simulink model "full_correlator"  (R2022a)
settings: Solver=VariableStepDiscrete  StartTime=0.0  StopTime=4000  RelTol=1e-3
libraries: hdlBasic x2638, hdlSSR x215, hdlDSPIP x4, xbsIndex_r4 x1, xps_library x1
(part 3 of 43)

== system full_correlator/Subsystem ==
  din : Inport
  vin : Inport  Port=2
  Concat : hdlBasic/Concat  num_inputs=8  XmcBlockStatus=1  maskContainerNames=group1  block_type=concat  block_config=sysgen:Concat_config
  Reinterpret : hdlBasic/Reinterpret  force_arith_type=on  arith_type=Unsigned  force_bin_pt=on  bin_pt=0  XmcBlockStatus=1  maskContainerNames=group1  block_type=reinterpret  block_config=sysgen:Reinterpret_config
  Scalar to Vector2 : hdlSSR/Scalar2Vector  Width=18  sg_ssr=8  block_type=scalar2vector_ssr  XmcBlockStatus=1  sg_ssr_prev=8  maskContainerNames=group1
  Time Division Demultiplexer2 : hdlBasic/Time Division Demultiplexer  frame_pattern=[1 1 1 1 1 1 1 1]  impl_style=Multiple Channel  vin=on  explicit_period=off  period=1  XmcBlockStatus=1  maskContainerNames=group2  block_type=tdd  block_config=sysgen:TDD_config
  Vector Reinterpret2 : hdlSSR/Vector Reinterpret  force_arith_type=on  arith_type="Signed  (2's comp)"  force_bin_pt=on  bin_pt=17  sg_ssr=8  block_type=reinterpret_ssr  XmcBlockStatus=1  sg_ssr_prev=8  maskContainerNames=group1
  dout : Outport
  vout : Outport  Port=2
  wires:
  Time Division Demultiplexer2/8 -> Concat/1
  Time Division Demultiplexer2/5 -> Concat/4
  Time Division Demultiplexer2/9 -> vout/1
  din/1 -> Reinterpret/1
  Time Division Demultiplexer2/3 -> Concat/6
  Reinterpret/1 -> Time Division Demultiplexer2/1
  Scalar to Vector2/1 -> Vector Reinterpret2/1
  Time Division Demultiplexer2/6 -> Concat/3
  Concat/1 -> Scalar to Vector2/1
  Time Division Demultiplexer2/7 -> Concat/2
  Time Division Demultiplexer2/4 -> Concat/5
  Time Division Demultiplexer2/2 -> Concat/7
  Vector Reinterpret2/1 -> dout/1
  vin/1 -> Time Division Demultiplexer2/2
  Time Division Demultiplexer2/1 -> Concat/8

== system full_correlator/Subsystem1 ==
  addr : Inport
  we : Inport  Port=2
  din : Inport  Port=3
  Concat{,1..3} (4 alike) : hdlBasic/Concat  num_inputs=2  XmcBlockStatus=1  maskContainerNames=group1  block_type=concat  block_config=sysgen:Concat_config
  Constant{2..5} (4 alike) : hdlBasic/Constant  const=0  gui_display_data_type=Fixed-point  arith_type=Unsigned  n_bits=56  bin_pt=0  preci_type=Single  exp_width=8  frac_width=24  explicit_period=off  period=1  XmcBlockStatus=1  maskContainerNames=tabcontainer1  block_type=constant  block_config=sysgen:Constant_config
  Terminator{7..10} (4 alike) : Terminator
  Vector Reinterpret : hdlSSR/Vector Reinterpret  force_arith_type=on  arith_type=Unsigned  force_bin_pt=on  bin_pt=0  sg_ssr=16  block_type=reinterpret_ssr  XmcBlockStatus=1  sg_ssr_prev=16  maskContainerNames=group1
  Vector to Scalar : hdlSSR/Vector2Scalar  sg_ssr=16  block_type=vector2scalar_ssr  XmcBlockStatus=1  sg_ssr_prev=16  maskContainerNames=group1
  bus_expand : Subsystem  AncestorBlock=casper_library_flow_control/bus_expand  mask(bus_expand){mode=divisions of equal size, outputNum=4, outputWidth=72, outputBinaryPt=0, outputArithmeticType=0, show_format=off, outputToWorkspace=off, variablePrefix=out, outputToModelAsWell=on}
      mask prompts: outputNum "Number of outputs:"; outputWidth "Output width:"; outputBinaryPt "Output binary point position:"; outputArithmeticType "Output arithmetic type (ufix=0, fix=1, bool=2):"; show_format "Print format string?"; outputToWorkspace "Output to workspace?"; variablePrefix "Variable name prefix:"; outputToModelAsWell "Output to model as well?"
      mask help:
      | Expands a 'bus' made using a bus_create or Xilinx
      | concat block.
      | The input will be divided into the specified number
      | of outputs with the specified arithmetic types.
      | Divisions are made from most significant bit.
      mask init: same as full_correlator/bus_expand
      settings: AttributesFormatString=4 outputs
      mask TypeOptions mode: divisions of equal size | divisions of arbitrary size
      mask Callback mode: %bus_expand_callback();
      mask Callback outputWidth: %bus_expand_callback();
      mask Callback outputToWorkspace: %bus_expand_callback();
  shared_bram : Subsystem  Tag=xps:bram  AncestorBlock=xps_library/Memory/shared_bram  mask{arith_type=Unsigned, addr_width=6, data_width=128, reg_prim_output=off, reg_core_output=off, optimization=Minimum_Area, data_bin_pt=0, init_vals=[0:2^10-1], sample_rate=1}
      mask prompts: arith_type "Output Data Type"; addr_width "Address width"; data_width "Data Width"; reg_prim_output "Register Primitive Output"; reg_core_output "Register Core Output"; data_bin_pt "Data Binary Point"; init_vals "Initial values (simulation only)"; sample_rate "Sample rate"
      mask init:
      | shared_bram_mask;
      mask TypeOptions arith_type: Unsigned | Signed  (2's comp)
      mask TypeOptions data_width: 8 | 16 | 32 | 64 | 128
      mask TypeOptions optimization: Minimum_Area | Low_Power
  shared_bram1 : Subsystem  Tag=xps:bram  AncestorBlock=xps_library/Memory/shared_bram  mask{arith_type=Unsigned, addr_width=6, data_width=128, reg_prim_output=off, reg_core_output=off, optimization=Minimum_Area, data_bin_pt=0, init_vals=[0:2^10-1], sample_rate=1}
      mask prompts: arith_type "Output Data Type"; addr_width "Address width"; data_width "Data Width"; reg_prim_output "Register Primitive Output"; reg_core_output "Register Core Output"; data_bin_pt "Data Binary Point"; init_vals "Initial values (simulation only)"; sample_rate "Sample rate"
      mask init:
      | shared_bram_mask;
      mask TypeOptions arith_type: Unsigned | Signed  (2's comp)
      mask TypeOptions data_width: 8 | 16 | 32 | 64 | 128
      mask TypeOptions optimization: Minimum_Area | Low_Power
  shared_bram2 : Subsystem  Tag=xps:bram  AncestorBlock=xps_library/Memory/shared_bram  mask{arith_type=Unsigned, addr_width=6, data_width=128, reg_prim_output=off, reg_core_output=off, optimization=Minimum_Area, data_bin_pt=0, init_vals=[0:2^10-1], sample_rate=1}
      mask prompts: arith_type "Output Data Type"; addr_width "Address width"; data_width "Data Width"; reg_prim_output "Register Primitive Output"; reg_core_output "Register Core Output"; data_bin_pt "Data Binary Point"; init_vals "Initial values (simulation only)"; sample_rate "Sample rate"
      mask init:
      | shared_bram_mask;
      mask TypeOptions arith_type: Unsigned | Signed  (2's comp)
      mask TypeOptions data_width: 8 | 16 | 32 | 64 | 128
      mask TypeOptions optimization: Minimum_Area | Low_Power
  shared_bram3 : Subsystem  Tag=xps:bram  AncestorBlock=xps_library/Memory/shared_bram  mask{arith_type=Unsigned, addr_width=6, data_width=128, reg_prim_output=off, reg_core_output=off, optimization=Minimum_Area, data_bin_pt=0, init_vals=[0:2^10-1], sample_rate=1}
      mask prompts: arith_type "Output Data Type"; addr_width "Address width"; data_width "Data Width"; reg_prim_output "Register Primitive Output"; reg_core_output "Register Core Output"; data_bin_pt "Data Binary Point"; init_vals "Initial values (simulation only)"; sample_rate "Sample rate"
      mask init:
      | shared_bram_mask;
      mask TypeOptions arith_type: Unsigned | Signed  (2's comp)
      mask TypeOptions data_width: 8 | 16 | 32 | 64 | 128
      mask TypeOptions optimization: Minimum_Area | Low_Power
  wires:
  Constant3/1 -> Concat1/2
  shared_bram1/1(data_out) -> Terminator8/1
  Constant5/1 -> Concat3/2
  addr/1 -> shared_bram/1(addr), shared_bram1/1(addr), shared_bram2/1(addr), shared_bram3/1(addr)
  shared_bram/1(data_out) -> Terminator7/1
  Constant2/1 -> Concat/2
  shared_bram3/1(data_out) -> Terminator10/1
  Concat1/1 -> shared_bram1/2(data_in)
  Constant4/1 -> Concat2/2
  din/1 -> Vector Reinterpret/1
  shared_bram2/1(data_out) -> Terminator9/1
  we/1 -> shared_bram/3(we), shared_bram1/3(we), shared_bram2/3(we), shared_bram3/3(we)
  Concat3/1 -> shared_bram3/2(data_in)
  Concat/1 -> shared_bram/2(data_in)
  Concat2/1 -> shared_bram2/2(data_in)
  Vector Reinterpret/1 -> Vector to Scalar/1
  Vector to Scalar/1 -> bus_expand/1(bus_in)
  bus_expand/1(msb_out4) -> Concat/1
  bus_expand/2(out3) -> Concat1/1
  bus_expand/3(out2) -> Concat2/1
  bus_expand/4(lsb_out1) -> Concat3/1

== system full_correlator/Subsystem2 ==
  addr : Inport
  we : Inport  Port=2
  din : Inport  Port=3
  Concat{,1..3} (4 alike) : hdlBasic/Concat  num_inputs=2  XmcBlockStatus=1  maskContainerNames=group1  block_type=concat  block_config=sysgen:Concat_config
  Constant{2..5} (4 alike) : hdlBasic/Constant  const=0  gui_display_data_type=Fixed-point  arith_type=Unsigned  n_bits=56  bin_pt=0  preci_type=Single  exp_width=8  frac_width=24  explicit_period=off  period=1  XmcBlockStatus=1  maskContainerNames=tabcontainer1  block_type=constant  block_config=sysgen:Constant_config
  Terminator{7..10} (4 alike) : Terminator
  Vector Reinterpret : hdlSSR/Vector Reinterpret  force_arith_type=on  arith_type=Unsigned  force_bin_pt=on  bin_pt=0  sg_ssr=16  block_type=reinterpret_ssr  XmcBlockStatus=1  sg_ssr_prev=16  maskContainerNames=group1
  Vector to Scalar : hdlSSR/Vector2Scalar  sg_ssr=16  block_type=vector2scalar_ssr  XmcBlockStatus=1  sg_ssr_prev=16  maskContainerNames=group1
  bus_expand : Subsystem  AncestorBlock=casper_library_flow_control/bus_expand  mask(bus_expand){mode=divisions of equal size, outputNum=4, outputWidth=72, outputBinaryPt=0, outputArithmeticType=0, show_format=off, outputToWorkspace=off, variablePrefix=out, outputToModelAsWell=on}
      mask prompts: outputNum "Number of outputs:"; outputWidth "Output width:"; outputBinaryPt "Output binary point position:"; outputArithmeticType "Output arithmetic type (ufix=0, fix=1, bool=2):"; show_format "Print format string?"; outputToWorkspace "Output to workspace?"; variablePrefix "Variable name prefix:"; outputToModelAsWell "Output to model as well?"
      mask help:
      | Expands a 'bus' made using a bus_create or Xilinx
      | concat block.
      | The input will be divided into the specified number
      | of outputs with the specified arithmetic types.
      | Divisions are made from most significant bit.
      mask init: same as full_correlator/bus_expand
      settings: AttributesFormatString=4 outputs
      mask TypeOptions mode: divisions of equal size | divisions of arbitrary size
      mask Callback mode: %bus_expand_callback();
      mask Callback outputWidth: %bus_expand_callback();
      mask Callback outputToWorkspace: %bus_expand_callback();
  shared_bram : Subsystem  Tag=xps:bram  AncestorBlock=xps_library/Memory/shared_bram  mask{arith_type=Unsigned, addr_width=6, data_width=128, reg_prim_output=off, reg_core_output=off, optimization=Minimum_Area, data_bin_pt=0, init_vals=[0:2^10-1], sample_rate=1}
      mask prompts: arith_type "Output Data Type"; addr_width "Address width"; data_width "Data Width"; reg_prim_output "Register Primitive Output"; reg_core_output "Register Core Output"; data_bin_pt "Data Binary Point"; init_vals "Initial values (simulation only)"; sample_rate "Sample rate"
      mask init:
      | shared_bram_mask;
      mask TypeOptions arith_type: Unsigned | Signed  (2's comp)
      mask TypeOptions data_width: 8 | 16 | 32 | 64 | 128
      mask TypeOptions optimization: Minimum_Area | Low_Power
  shared_bram1 : Subsystem  Tag=xps:bram  AncestorBlock=xps_library/Memory/shared_bram  mask{arith_type=Unsigned, addr_width=6, data_width=128, reg_prim_output=off, reg_core_output=off, optimization=Minimum_Area, data_bin_pt=0, init_vals=[0:2^10-1], sample_rate=1}
      mask prompts: arith_type "Output Data Type"; addr_width "Address width"; data_width "Data Width"; reg_prim_output "Register Primitive Output"; reg_core_output "Register Core Output"; data_bin_pt "Data Binary Point"; init_vals "Initial values (simulation only)"; sample_rate "Sample rate"
      mask init:
      | shared_bram_mask;
      mask TypeOptions arith_type: Unsigned | Signed  (2's comp)
      mask TypeOptions data_width: 8 | 16 | 32 | 64 | 128
      mask TypeOptions optimization: Minimum_Area | Low_Power
  shared_bram2 : Subsystem  Tag=xps:bram  AncestorBlock=xps_library/Memory/shared_bram  mask{arith_type=Unsigned, addr_width=6, data_width=128, reg_prim_output=off, reg_core_output=off, optimization=Minimum_Area, data_bin_pt=0, init_vals=[0:2^10-1], sample_rate=1}
      mask prompts: arith_type "Output Data Type"; addr_width "Address width"; data_width "Data Width"; reg_prim_output "Register Primitive Output"; reg_core_output "Register Core Output"; data_bin_pt "Data Binary Point"; init_vals "Initial values (simulation only)"; sample_rate "Sample rate"
      mask init:
      | shared_bram_mask;
      mask TypeOptions arith_type: Unsigned | Signed  (2's comp)
      mask TypeOptions data_width: 8 | 16 | 32 | 64 | 128
      mask TypeOptions optimization: Minimum_Area | Low_Power
  shared_bram3 : Subsystem  Tag=xps:bram  AncestorBlock=xps_library/Memory/shared_bram  mask{arith_type=Unsigned, addr_width=6, data_width=128, reg_prim_output=off, reg_core_output=off, optimization=Minimum_Area, data_bin_pt=0, init_vals=[0:2^10-1], sample_rate=1}
      mask prompts: arith_type "Output Data Type"; addr_width "Address width"; data_width "Data Width"; reg_prim_output "Register Primitive Output"; reg_core_output "Register Core Output"; data_bin_pt "Data Binary Point"; init_vals "Initial values (simulation only)"; sample_rate "Sample rate"
      mask init:
      | shared_bram_mask;
      mask TypeOptions arith_type: Unsigned | Signed  (2's comp)
      mask TypeOptions data_width: 8 | 16 | 32 | 64 | 128
      mask TypeOptions optimization: Minimum_Area | Low_Power
  wires:
  Constant3/1 -> Concat1/2
  shared_bram1/1(data_out) -> Terminator8/1
  Constant5/1 -> Concat3/2
  addr/1 -> shared_bram/1(addr), shared_bram1/1(addr), shared_bram2/1(addr), shared_bram3/1(addr)
  shared_bram/1(data_out) -> Terminator7/1
  Constant2/1 -> Concat/2
  shared_bram3/1(data_out) -> Terminator10/1
  Concat1/1 -> shared_bram1/2(data_in)
  Constant4/1 -> Concat2/2
  din/1 -> Vector Reinterpret/1
  shared_bram2/1(data_out) -> Terminator9/1
  we/1 -> shared_bram/3(we), shared_bram1/3(we), shared_bram2/3(we), shared_bram3/3(we)
  Concat3/1 -> shared_bram3/2(data_in)
  Concat/1 -> shared_bram/2(data_in)
  Concat2/1 -> shared_bram2/2(data_in)
  Vector Reinterpret/1 -> Vector to Scalar/1
  Vector to Scalar/1 -> bus_expand/1(bus_in)
  bus_expand/1(msb_out4) -> Concat/1
  bus_expand/2(out3) -> Concat1/1
  bus_expand/3(out2) -> Concat2/1
  bus_expand/4(lsb_out1) -> Concat3/1

== system full_correlator/Subsystem3 ==
  din : Inport
  vin : Inport  Port=2
  Concat : hdlBasic/Concat  num_inputs=8  XmcBlockStatus=1  maskContainerNames=group1  block_type=concat  block_config=sysgen:Concat_config
  Reinterpret : hdlBasic/Reinterpret  force_arith_type=on  arith_type=Unsigned  force_bin_pt=on  bin_pt=0  XmcBlockStatus=1  maskContainerNames=group1  block_type=reinterpret  block_config=sysgen:Reinterpret_config
  Scalar to Vector2 : hdlSSR/Scalar2Vector  Width=18  sg_ssr=8  block_type=scalar2vector_ssr  XmcBlockStatus=1  sg_ssr_prev=8  maskContainerNames=group1
  Time Division Demultiplexer2 : hdlBasic/Time Division Demultiplexer  frame_pattern=[1 1 1 1 1 1 1 1]  impl_style=Multiple Channel  vin=on  explicit_period=off  period=1  XmcBlockStatus=1  maskContainerNames=group2  block_type=tdd  block_config=sysgen:TDD_config
  Vector Reinterpret2 : hdlSSR/Vector Reinterpret  force_arith_type=on  arith_type="Signed  (2's comp)"  force_bin_pt=on  bin_pt=17  sg_ssr=8  block_type=reinterpret_ssr  XmcBlockStatus=1  sg_ssr_prev=8  maskContainerNames=group1
  dout : Outport
  vout : Outport  Port=2
  wires:
  Time Division Demultiplexer2/8 -> Concat/1
  Time Division Demultiplexer2/5 -> Concat/4
  Time Division Demultiplexer2/9 -> vout/1
  din/1 -> Reinterpret/1
  Time Division Demultiplexer2/3 -> Concat/6
  Reinterpret/1 -> Time Division Demultiplexer2/1
  Scalar to Vector2/1 -> Vector Reinterpret2/1
  Time Division Demultiplexer2/6 -> Concat/3
  Concat/1 -> Scalar to Vector2/1
  Time Division Demultiplexer2/7 -> Concat/2
  Time Division Demultiplexer2/4 -> Concat/5
  Time Division Demultiplexer2/2 -> Concat/7
  Vector Reinterpret2/1 -> dout/1
  vin/1 -> Time Division Demultiplexer2/2
  Time Division Demultiplexer2/1 -> Concat/8

== system full_correlator/Subsystem4 ==
  IN : Inport
  Scalar to Vector2 : hdlSSR/Scalar2Vector  Width=18  sg_ssr=8  block_type=scalar2vector_ssr  XmcBlockStatus=1  sg_ssr_prev=8  maskContainerNames=group1
  Up Sample2 : hdlBasic/Up Sample  sample_ratio=8  copy_samples=on  en=off  latency=1  XmcBlockStatus=1  maskContainerNames=group1  block_type=usamp  block_config=sysgen:Upsample_config
  Vector Reinterpret2 : hdlSSR/Vector Reinterpret  force_arith_type=on  arith_type=Unsigned  force_bin_pt=on  bin_pt=0  sg_ssr=8  block_type=reinterpret_ssr  XmcBlockStatus=1  sg_ssr_prev=8  maskContainerNames=group1
  Vector Reinterpret3 : hdlSSR/Vector Reinterpret  force_arith_type=on  arith_type="Signed  (2's comp)"  force_bin_pt=on  bin_pt=17  sg_ssr=8  block_type=reinterpret_ssr  XmcBlockStatus=1  sg_ssr_prev=8  maskContainerNames=group1
  Vector to Scalar1 : hdlSSR/Vector2Scalar  sg_ssr=8  block_type=vector2scalar_ssr  XmcBlockStatus=1  sg_ssr_prev=8  maskContainerNames=group1
  OUT : Outport
  wires:
  Scalar to Vector2/1 -> Vector Reinterpret3/1
  Vector Reinterpret3/1 -> OUT/1
  Vector Reinterpret2/1 -> Vector to Scalar1/1
  Vector to Scalar1/1 -> Up Sample2/1
  Up Sample2/1 -> Scalar to Vector2/1
  IN/1 -> Vector Reinterpret2/1

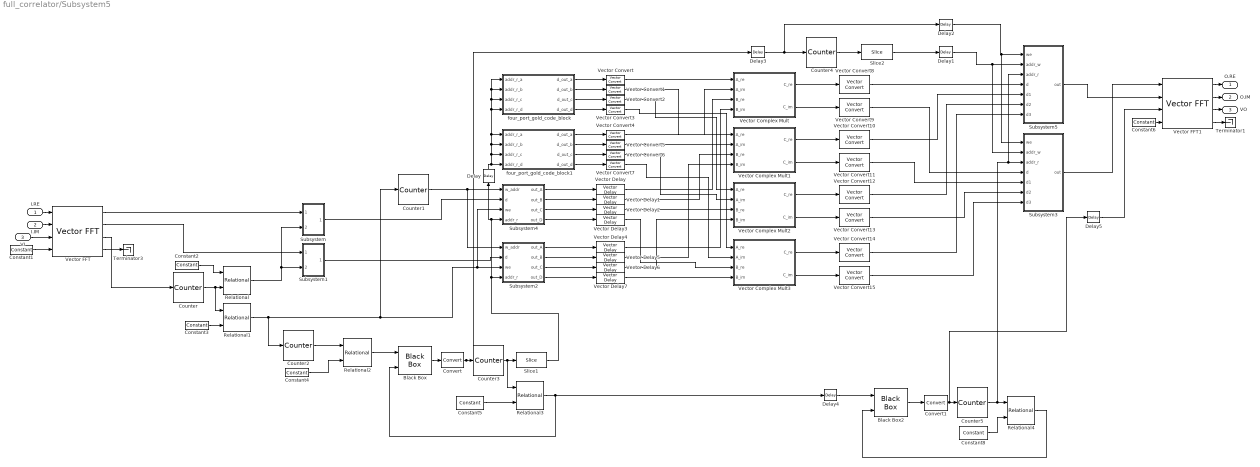
== system full_correlator/Subsystem5 ==
  I.RE : Inport
  I.IM : Inport  Port=2
  VI : Inport  Port=3
  Black Box : hdlBasic/Black Box  init_code=sr_flip_flop_config  sim_method=Vivado Simulator  verbose=off  XmcBlockStatus=1  maskContainerNames=group1  block_type=blackbox2  block_config=sysgen:black_box_config
  Black Box2 : hdlBasic/Black Box  init_code=sr_flip_flop_config  sim_method=Vivado Simulator  verbose=off  XmcBlockStatus=1  maskContainerNames=group1  block_type=blackbox2  block_config=sysgen:black_box_config
  Constant1 : hdlBasic/Constant  const=1023  gui_display_data_type=Fixed-point  arith_type=Unsigned  n_bits=10  bin_pt=0  preci_type=Single  exp_width=8  frac_width=24  explicit_period=on  period=1  XmcBlockStatus=1  maskContainerNames=tabcontainer1  block_type=constant  block_config=sysgen:Constant_config
  Constant2 : hdlBasic/Constant  const=0  gui_display_data_type=Fixed-point  arith_type=Unsigned  n_bits=1  bin_pt=0  preci_type=Single  exp_width=8  frac_width=24  explicit_period=on  period=1  XmcBlockStatus=1  maskContainerNames=tabcontainer1  block_type=constant  block_config=sysgen:Constant_config
  Constant3 : hdlBasic/Constant  const=1  gui_display_data_type=Fixed-point  arith_type=Unsigned  n_bits=1  bin_pt=0  preci_type=Single  exp_width=8  frac_width=24  explicit_period=on  period=1  XmcBlockStatus=1  maskContainerNames=tabcontainer1  block_type=constant  block_config=sysgen:Constant_config
  Constant4 : hdlBasic/Constant  const=63  gui_display_data_type=Fixed-point  arith_type=Unsigned  n_bits=6  bin_pt=0  preci_type=Single  exp_width=8  frac_width=24  explicit_period=on  period=1  XmcBlockStatus=1  maskContainerNames=tabcontainer1  block_type=constant  block_config=sysgen:Constant_config
  Constant5 : hdlBasic/Constant  const=126  gui_display_data_type=Fixed-point  arith_type=Unsigned  n_bits=7  bin_pt=0  preci_type=Single  exp_width=8  frac_width=24  explicit_period=on  period=1  XmcBlockStatus=1  maskContainerNames=tabcontainer1  block_type=constant  block_config=sysgen:Constant_config
  Constant6 : hdlBasic/Constant  const=1023  gui_display_data_type=Fixed-point  arith_type=Unsigned  n_bits=10  bin_pt=0  preci_type=Single  exp_width=8  frac_width=24  explicit_period=on  period=1  XmcBlockStatus=1  maskContainerNames=tabcontainer1  block_type=constant  block_config=sysgen:Constant_config
  Constant8 : hdlBasic/Constant  const=62  gui_display_data_type=Fixed-point  arith_type=Unsigned  n_bits=6  bin_pt=0  preci_type=Single  exp_width=8  frac_width=24  explicit_period=on  period=1  XmcBlockStatus=1  maskContainerNames=tabcontainer1  block_type=constant  block_config=sysgen:Constant_config
  Convert : hdlBasic/Convert  gui_display_data_type=Boolean  arith_type=Boolean  n_bits=16  bin_pt=14  float_type=Single  exp_bits=8  fraction_bits=24  quantization=Truncate  overflow=Wrap  en=off  latency=0  pipeline=off  XmcBlockStatus=1  maskContainerNames=group2  block_type=convert  block_config=sysgen:Convert_config  block_width=595  block_height=885
  Convert1 : hdlBasic/Convert  gui_display_data_type=Boolean  arith_type=Boolean  n_bits=16  bin_pt=14  float_type=Single  exp_bits=8  fraction_bits=24  quantization=Truncate  overflow=Wrap  en=off  latency=0  pipeline=off  XmcBlockStatus=1  maskContainerNames=group2  block_type=convert  block_config=sysgen:Convert_config  block_width=595  block_height=885
  Counter : hdlBasic/Counter  cnt_type=Free running  cnt_to=Inf  operation=Up  start_count=0  cnt_by_val=1  arith_type=Unsigned  n_bits=1  bin_pt=0  load_pin=off  rst=off  en=on  explicit_period=Explicit  period=1  use_behavioral_HDL=off  implementation=Fabric  XmcBlockStatus=1  maskContainerNames=group1  block_type=counter  block_config=sysgen:Counter_config  block_width=531  block_height=1023
  Counter1 : hdlBasic/Counter  cnt_type=Free running  cnt_to=Inf  operation=Up  start_count=0  cnt_by_val=1  arith_type=Unsigned  n_bits=6  bin_pt=0  load_pin=off  rst=off  en=on  explicit_period=Explicit  period=1  use_behavioral_HDL=off  implementation=Fabric  XmcBlockStatus=1  maskContainerNames=group1  block_type=counter  block_config=sysgen:Counter_config  block_width=531  block_height=1023
  Counter2 : hdlBasic/Counter  cnt_type=Free running  cnt_to=Inf  operation=Up  start_count=0  cnt_by_val=1  arith_type=Unsigned  n_bits=6  bin_pt=0  load_pin=off  rst=off  en=on  explicit_period=Explicit  period=1  use_behavioral_HDL=off  implementation=Fabric  XmcBlockStatus=1  maskContainerNames=group1  block_type=counter  block_config=sysgen:Counter_config  block_width=531  block_height=1023
  Counter3 : hdlBasic/Counter  cnt_type=Free running  cnt_to=Inf  operation=Up  start_count=0  cnt_by_val=1  arith_type=Unsigned  n_bits=7  bin_pt=0  load_pin=off  rst=off  en=on  explicit_period=Explicit  period=1  use_behavioral_HDL=off  implementation=Fabric  XmcBlockStatus=1  maskContainerNames=group1  block_type=counter  block_config=sysgen:Counter_config  block_width=531  block_height=1023
  Counter4 : hdlBasic/Counter  cnt_type=Free running  cnt_to=Inf  operation=Up  start_count=0  cnt_by_val=1  arith_type=Unsigned  n_bits=7  bin_pt=0  load_pin=off  rst=off  en=on  explicit_period=Explicit  period=1  use_behavioral_HDL=off  implementation=Fabric  XmcBlockStatus=1  maskContainerNames=group1  block_type=counter  block_config=sysgen:Counter_config  block_width=531  block_height=1023
  Counter5 : hdlBasic/Counter  cnt_type=Free running  cnt_to=Inf  operation=Up  start_count=0  cnt_by_val=1  arith_type=Unsigned  n_bits=6  bin_pt=0  load_pin=off  rst=off  en=on  explicit_period=Explicit  period=1  use_behavioral_HDL=off  implementation=Fabric  XmcBlockStatus=1  maskContainerNames=group1  block_type=counter  block_config=sysgen:Counter_config  block_width=531  block_height=1023
  Delay : hdlBasic/Delay  rst=off  en=off  latency=2  reg_retiming=off  XmcBlockStatus=1  maskContainerNames=group1  block_type=delay  block_config=sysgen:Delay_config
  Delay1 : hdlBasic/Delay  rst=off  en=off  latency=1  reg_retiming=off  XmcBlockStatus=1  maskContainerNames=group1  block_type=delay  block_config=sysgen:Delay_config
  Delay2 : hdlBasic/Delay  rst=off  en=off  latency=1  reg_retiming=off  XmcBlockStatus=1  maskContainerNames=group1  block_type=delay  block_config=sysgen:Delay_config
  Delay3 : hdlBasic/Delay  rst=off  en=off  latency=10  reg_retiming=off  XmcBlockStatus=1  maskContainerNames=group1  block_type=delay  block_config=sysgen:Delay_config
  Delay4 : hdlBasic/Delay  rst=off  en=off  latency=11  reg_retiming=off  XmcBlockStatus=1  maskContainerNames=group1  block_type=delay  block_config=sysgen:Delay_config
  Delay5 : hdlBasic/Delay  rst=off  en=off  latency=6  reg_retiming=off  XmcBlockStatus=1  maskContainerNames=group1  block_type=delay  block_config=sysgen:Delay_config
  Relational : hdlBasic/Relational  mode=a=b  op_type=Bool  en=off  latency=0  XmcBlockStatus=1  maskContainerNames=tabcontainer1  block_type=relational  block_config=sysgen:Relational_config
  Relational1 : hdlBasic/Relational  mode=a=b  op_type=Bool  en=off  latency=0  XmcBlockStatus=1  maskContainerNames=tabcontainer1  block_type=relational  block_config=sysgen:Relational_config
  Relational2 : hdlBasic/Relational  mode=a=b  op_type=Bool  en=off  latency=1  XmcBlockStatus=1  maskContainerNames=tabcontainer1  block_type=relational  block_config=sysgen:Relational_config
  Relational3 : hdlBasic/Relational  mode=a=b  op_type=Bool  en=off  latency=1  XmcBlockStatus=1  maskContainerNames=tabcontainer1  block_type=relational  block_config=sysgen:Relational_config
  Relational4 : hdlBasic/Relational  mode=a=b  op_type=Bool  en=off  latency=1  XmcBlockStatus=1  maskContainerNames=tabcontainer1  block_type=relational  block_config=sysgen:Relational_config
  Slice1 : hdlBasic/Slice  nbits=4  boolean_output=off  mode=Upper Bit Location + Width  bit1=0  base1=MSB of Input  bit0=0  base0=LSB of Input  XmcBlockStatus=1  maskContainerNames=group1  block_type=slice  block_config=sysgen:Slice_config
  Slice2 : hdlBasic/Slice  nbits=4  boolean_output=off  mode=Upper Bit Location + Width  bit1=0  base1=MSB of Input  bit0=0  base0=LSB of Input  XmcBlockStatus=1  maskContainerNames=group1  block_type=slice  block_config=sysgen:Slice_config
  Subsystem : Subsystem
  Subsystem1 : Subsystem
  Subsystem2 : Subsystem
  Subsystem3 : Subsystem
  Subsystem4 : Subsystem
  Subsystem5 : Subsystem
  Terminator1 : Terminator
  Terminator3 : Terminator
  Vector Complex Mult : Subsystem  LoadFcn=obj = XmcLoadGUI(gcbh); obj.loadGUI();  mask(Xilinx Vector Complex Multiplier Block){sg_ssr=16, use_synth_mdl=off, sg_icon_stat=, sg_mask_display=|, block_version=, block_type=cmplxmult_ssr, XmcBlockStatus=1, sg_ssr_prev=16, SD={'sg_ssr'=>'Int','use_synth_mdl'=>'Int','xinports'=>'DoubleVector','xoutports'=>'DoubleVector','block_type'=>'String'}, maskContainerNames=group1}
      mask sg_mask_display=|
      | xmcDrawHDLBlockIcon();
      | fprintf('','COMMENT: begin icon text');
      |
      | color('black');port_label('input',1,' A_re');
      | color('black');port_label('input',2,' A_im');
      | color('black');port_label('input',3,' B_re');
      | color('black');port_label('input',4,' B_im');
      |
      | color('black');disp('25x18 signed \newline Latency = 6','texmode','on');
      |
      | color('black');port_label('output',1,'C_re');
      | color('black');port_label('output',2,'C_im');
      mask prompts: sg_ssr "SSR"; use_synth_mdl "Use Synthesizable model"
      mask help: Vector Complex Multiplier block supports complext multiplication for input of vector types.
      mask init:
      | this = gcb;
      | xlSSRParamEvaluation;
      | isElabReq = xlSSRIsElabReq(this,sg_ssr);
      | if (sg_ssr ~= sg_ssr_prev || isElabReq)
      |     try
      |         xlSSRCmplxMult;
      |         set_param(this,'sg_ssr_prev',num2str(sg_ssr));
      |     catch ME
      |         disp(['Error while updating -> ' this])
      |         disp(ME.message)
      |     end
      | else
      |    xlSSRCmplxMultInitGUI;
      | end
      mask Help: helpview(vmcHelp)
      mask Callback sg_ssr: obj = XmcUpdateGUI(gcbh, @xlmagicenablement, -1); obj.updateGUI()
      mask Callback use_synth_mdl: obj = XmcUpdateGUI(gcbh, @xlmagicenablement, -1); obj.updateGUI()
      mask TypeOptions maskContainerNames: group1 | infoedit | tabcontainer1 | basictab | Impltab
      mask DialogControl DescGroupVar Prompt: Vector Complex Mult
      mask DialogControl infoedit Prompt: The Vector Complex Multiplier block supports multiplication of two complex input vectors.
      mask DialogControl basictab Prompt: Basic
      mask DialogControl Impltab Prompt: Implementation
      mask Display:
      | xmcDrawHDLBlockIcon();
      | fprintf('','COMMENT: begin icon text');
      | 
      | color('black');port_label('input',1,' A_re');
      | color('black');port_label('input',2,' A_im');
      | color('black');port_label('input',3,' B_re');
      | color('black');port_label('input',4,' B_im');
      | 
      | color('black');disp('25x18 signed \newline Latency = 6','texmode','on');
      | 
      | color('black');port_label('output',1,'C_re');
      | color('black');port_label('output',2,'C_im');
  Vector Complex Mult1 : Subsystem  LoadFcn=obj = XmcLoadGUI(gcbh); obj.loadGUI();  mask(Xilinx Vector Complex Multiplier Block){sg_ssr=16, use_synth_mdl=off, sg_icon_stat=, sg_mask_display=|, block_version=, block_type=cmplxmult_ssr, XmcBlockStatus=1, sg_ssr_prev=16, SD={'sg_ssr'=>'Int','use_synth_mdl'=>'Int','xinports'=>'DoubleVector','xoutports'=>'DoubleVector','block_type'=>'String'}, maskContainerNames=group1}
      mask sg_mask_display=|
      | xmcDrawHDLBlockIcon();
      | fprintf('','COMMENT: begin icon text');
      |
      | color('black');port_label('input',1,' A_re');
      | color('black');port_label('input',2,' A_im');
      | color('black');port_label('input',3,' B_re');
      | color('black');port_label('input',4,' B_im');
      |
      | color('black');disp('25x18 signed \newline Latency = 6','texmode','on');
      |
      | color('black');port_label('output',1,'C_re');
      | color('black');port_label('output',2,'C_im');
      mask prompts: sg_ssr "SSR"; use_synth_mdl "Use Synthesizable model"
      mask help: Vector Complex Multiplier block supports complext multiplication for input of vector types.
      mask init: same as full_correlator/Subsystem5/Vector Complex Mult
      mask Help: helpview(vmcHelp)
      mask Callback sg_ssr: obj = XmcUpdateGUI(gcbh, @xlmagicenablement, -1); obj.updateGUI()
      mask Callback use_synth_mdl: obj = XmcUpdateGUI(gcbh, @xlmagicenablement, -1); obj.updateGUI()
      mask TypeOptions maskContainerNames: group1 | infoedit | tabcontainer1 | basictab | Impltab
      mask DialogControl DescGroupVar Prompt: Vector Complex Mult
      mask DialogControl infoedit Prompt: The Vector Complex Multiplier block supports multiplication of two complex input vectors.
      mask DialogControl basictab Prompt: Basic
      mask DialogControl Impltab Prompt: Implementation
      mask Display:
      | xmcDrawHDLBlockIcon();
      | fprintf('','COMMENT: begin icon text');
      | 
      | color('black');port_label('input',1,' A_re');
      | color('black');port_label('input',2,' A_im');
      | color('black');port_label('input',3,' B_re');
      | color('black');port_label('input',4,' B_im');
      | 
      | color('black');disp('25x18 signed \newline Latency = 6','texmode','on');
      | 
      | color('black');port_label('output',1,'C_re');
      | color('black');port_label('output',2,'C_im');
  Vector Complex Mult2 : Subsystem  LoadFcn=obj = XmcLoadGUI(gcbh); obj.loadGUI();  mask(Xilinx Vector Complex Multiplier Block){sg_ssr=16, use_synth_mdl=off, sg_icon_stat=, sg_mask_display=|, block_version=, block_type=cmplxmult_ssr, XmcBlockStatus=1, sg_ssr_prev=16, SD={'sg_ssr'=>'Int','use_synth_mdl'=>'Int','xinports'=>'DoubleVector','xoutports'=>'DoubleVector','block_type'=>'String'}, maskContainerNames=group1}
      mask sg_mask_display=|
      | xmcDrawHDLBlockIcon();
      | fprintf('','COMMENT: begin icon text');
      |
      | color('black');port_label('input',1,' A_re');
      | color('black');port_label('input',2,' A_im');
      | color('black');port_label('input',3,' B_re');
      | color('black');port_label('input',4,' B_im');
      |
      | color('black');disp('25x18 signed \newline Latency = 6','texmode','on');
      |
      | color('black');port_label('output',1,'C_re');
      | color('black');port_label('output',2,'C_im');
      mask prompts: sg_ssr "SSR"; use_synth_mdl "Use Synthesizable model"
      mask help: Vector Complex Multiplier block supports complext multiplication for input of vector types.
      mask init: same as full_correlator/Subsystem5/Vector Complex Mult
      mask Help: helpview(vmcHelp)
      mask Callback sg_ssr: obj = XmcUpdateGUI(gcbh, @xlmagicenablement, -1); obj.updateGUI()
      mask Callback use_synth_mdl: obj = XmcUpdateGUI(gcbh, @xlmagicenablement, -1); obj.updateGUI()
      mask TypeOptions maskContainerNames: group1 | infoedit | tabcontainer1 | basictab | Impltab
      mask DialogControl DescGroupVar Prompt: Vector Complex Mult
      mask DialogControl infoedit Prompt: The Vector Complex Multiplier block supports multiplication of two complex input vectors.
      mask DialogControl basictab Prompt: Basic
      mask DialogControl Impltab Prompt: Implementation
      mask Display:
      | xmcDrawHDLBlockIcon();
      | fprintf('','COMMENT: begin icon text');
      | 
      | color('black');port_label('input',1,' A_re');
      | color('black');port_label('input',2,' A_im');
      | color('black');port_label('input',3,' B_re');
      | color('black');port_label('input',4,' B_im');
      | 
      | color('black');disp('25x18 signed \newline Latency = 6','texmode','on');
      | 
      | color('black');port_label('output',1,'C_re');
      | color('black');port_label('output',2,'C_im');
  Vector Complex Mult3 : Subsystem  LoadFcn=obj = XmcLoadGUI(gcbh); obj.loadGUI();  mask(Xilinx Vector Complex Multiplier Block){sg_ssr=16, use_synth_mdl=off, sg_icon_stat=, sg_mask_display=|, block_version=, block_type=cmplxmult_ssr, XmcBlockStatus=1, sg_ssr_prev=16, SD={'sg_ssr'=>'Int','use_synth_mdl'=>'Int','xinports'=>'DoubleVector','xoutports'=>'DoubleVector','block_type'=>'String'}, maskContainerNames=group1}
      mask sg_mask_display=|
      | xmcDrawHDLBlockIcon();
      | fprintf('','COMMENT: begin icon text');
      |
      | color('black');port_label('input',1,' A_re');
      | color('black');port_label('input',2,' A_im');
      | color('black');port_label('input',3,' B_re');
      | color('black');port_label('input',4,' B_im');
      |
      | color('black');disp('25x18 signed \newline Latency = 6','texmode','on');
      |
      | color('black');port_label('output',1,'C_re');
      | color('black');port_label('output',2,'C_im');
      mask prompts: sg_ssr "SSR"; use_synth_mdl "Use Synthesizable model"
      mask help: Vector Complex Multiplier block supports complext multiplication for input of vector types.
      mask init: same as full_correlator/Subsystem5/Vector Complex Mult
      mask Help: helpview(vmcHelp)
      mask Callback sg_ssr: obj = XmcUpdateGUI(gcbh, @xlmagicenablement, -1); obj.updateGUI()
      mask Callback use_synth_mdl: obj = XmcUpdateGUI(gcbh, @xlmagicenablement, -1); obj.updateGUI()
      mask TypeOptions maskContainerNames: group1 | infoedit | tabcontainer1 | basictab | Impltab
      mask DialogControl DescGroupVar Prompt: Vector Complex Mult
      mask DialogControl infoedit Prompt: The Vector Complex Multiplier block supports multiplication of two complex input vectors.
      mask DialogControl basictab Prompt: Basic
      mask DialogControl Impltab Prompt: Implementation
      mask Display:
      | xmcDrawHDLBlockIcon();
      | fprintf('','COMMENT: begin icon text');
      | 
      | color('black');port_label('input',1,' A_re');
      | color('black');port_label('input',2,' A_im');
      | color('black');port_label('input',3,' B_re');
      | color('black');port_label('input',4,' B_im');
      | 
      | color('black');disp('25x18 signed \newline Latency = 6','texmode','on');
      | 
      | color('black');port_label('output',1,'C_re');
      | color('black');port_label('output',2,'C_im');
  Vector Convert{,1..7} (8 alike) : hdlSSR/Vector Convert  gui_display_data_type=Fixed-point  arith_type=Signed (2's comp)  n_bits=26  bin_pt=17  float_type=Single  exp_bits=8  fraction_bits=24  quantization=Truncate  overflow=Wrap  en=off  sg_latency=1  sg_ssr=16  pipeline=off  block_type=convert_ssr  XmcBlockStatus=1  sg_ssr_prev=16  maskContainerNames=group2
  Vector Convert{8..15} (8 alike) : hdlSSR/Vector Convert  gui_display_data_type=Fixed-point  arith_type=Signed (2's comp)  n_bits=18  bin_pt=17  float_type=Single  exp_bits=8  fraction_bits=24  quantization=Truncate  overflow=Wrap  en=off  sg_latency=1  sg_ssr=16  pipeline=off  block_type=convert_ssr  XmcBlockStatus=1  sg_ssr_prev=16  maskContainerNames=group2
  Vector Delay{,1..7} (8 alike) : hdlSSR/Vector Delay  rst=off  en=off  vectorize_en=off  sg_latency=1  sg_ssr=16  reg_retiming=off  block_type=delay_ssr  XmcBlockStatus=1  sg_ssr_prev=16  maskContainerNames=group1
  Vector FFT : hdlSSR/Vector FFT  N=1024  n_bits=18  bin_pt=17  bram_threshold=258  sg_ssr=8  block_type=fft_ssr  W_high=1  W_low=-17  XmcBlockStatus=1  sg_ssr_prev=8  maskContainerNames=group3
  Vector FFT1 : hdlSSR/Vector FFT  N=1024  n_bits=18  bin_pt=17  bram_threshold=258  sg_ssr=16  block_type=fft_ssr  W_high=1  W_low=-17  XmcBlockStatus=1  sg_ssr_prev=16  maskContainerNames=group3
  four_port_gold_code_block : Subsystem
  four_port_gold_code_block1 : Subsystem
  O.RE : Outport
  O.IM : Outport  Port=2
  VO : Outport  Port=3
  wires:
  Subsystem5/1(out) -> Vector FFT1/2
  Subsystem2/3(out_C) -> Vector Delay6/1
  Vector Complex Mult1/1(C_re) -> Vector Convert10/1
  Black Box2/1 -> Convert1/1
  Vector Delay5/1 -> Vector Complex Mult1/4(B_im)
  Vector Complex Mult2/1(C_re) -> Vector Convert12/1
  Vector Convert9/1 -> Subsystem3/4(d)
  Vector Convert/1 -> Vector Complex Mult/1(A_re)
  Vector Convert15/1 -> Subsystem3/7(d3)
  Vector Convert14/1 -> Subsystem5/7(d3)
  Subsystem2/2(out_B) -> Vector Delay5/1
  Vector Convert13/1 -> Subsystem3/6(d2)
  Vector FFT1/4 -> Terminator1/1
  Subsystem4/2(out_B) -> Vector Delay1/1
  Delay2/1 -> Subsystem5/1(we), Subsystem3/1(we)
  Vector Convert8/1 -> Subsystem5/4(d)
  Vector Complex Mult/1(C_re) -> Vector Convert8/1
  Vector Complex Mult/2(C_im) -> Vector Convert9/1
  Delay4/1 -> Black Box2/1
  Vector Delay1/1 -> Vector Complex Mult1/3(B_re)
  Vector FFT/1 -> Subsystem/1(din)
  four_port_gold_code_block/3(d_out_c) -> Vector Convert2/1
  four_port_gold_code_block1/1(d_out_a) -> Vector Convert4/1
  VI/1 -> Vector FFT/3
  Vector Complex Mult2/2(C_im) -> Vector Convert13/1
  Vector Complex Mult3/2(C_im) -> Vector Convert15/1
  Vector Convert11/1 -> Subsystem3/5(d1)
  Vector Delay2/1 -> Vector Complex Mult2/3(B_re)
  Subsystem/1(out) -> Subsystem4/2(d)
  Vector Complex Mult3/1(C_re) -> Vector Convert14/1
  Subsystem4/3(out_C) -> Vector Delay2/1
  Relational3/1 -> Black Box/2, Delay4/1
  Delay5/1 -> Vector FFT1/3
  Constant8/1 -> Relational4/2
  Relational2/1 -> Black Box/1
  Vector Convert1/1 -> Vector Complex Mult1/1(A_re)
  Vector Delay6/1 -> Vector Complex Mult2/4(B_im)
  Counter3/1 -> Slice1/1, Relational3/1
  Subsystem2/1(out_A) -> Vector Delay4/1
  Delay3/1 -> Delay2/1, Counter4/1
  Vector Complex Mult1/2(C_im) -> Vector Convert11/1
  Vector Delay4/1 -> Vector Complex Mult/4(B_im)
  Delay/1 -> four_port_gold_code_block1/4(addr_r_d), four_port_gold_code_block1/3(addr_r_c), four_port_gold_code_block1/2(addr_r_b), four_port_gold_code_block1/1(addr_r_a), four_port_gold_code_block/4(addr_r_d), four_port_gold_code_block/3(addr_r_c), four_port_gold_code_block/2(addr_r_b), four_port_gold_code_block/1(addr_r_a)
  Vector FFT1/2 -> O.IM/1
  Convert/1 -> Delay3/1, Counter3/1
  I.IM/1 -> Vector FFT/2
  Vector Delay/1 -> Vector Complex Mult/3(B_re)
  four_port_gold_code_block/1(d_out_a) -> Vector Convert/1
  Subsystem2/4(out_D) -> Vector Delay7/1
  Vector FFT1/3 -> VO/1
  Vector Convert5/1 -> Vector Complex Mult1/2(A_im)
  Constant3/1 -> Relational1/2
  Vector FFT/2 -> Subsystem1/1(din)
  Vector FFT1/1 -> O.RE/1
  Counter5/1 -> Subsystem5/3(addr_r), Subsystem3/3(addr_r), Relational4/1
  Vector Delay3/1 -> Vector Complex Mult3/3(B_re)
  four_port_gold_code_block1/4(d_out_d) -> Vector Convert7/1
  Counter1/1 -> Subsystem2/1(w_addr), Subsystem4/1(w_addr)
  Vector Delay7/1 -> Vector Complex Mult3/4(B_im)
  Subsystem4/4(out_D) -> Vector Delay3/1
  Black Box/1 -> Convert/1
  Delay1/1 -> Subsystem5/2(addr_w), Subsystem3/2(addr_w)
  Vector FFT/4 -> Terminator3/1
  Vector Convert12/1 -> Subsystem5/6(d2)
  Vector FFT/3 -> Counter/1
  Relational1/1 -> Subsystem2/3(we), Subsystem4/3(we), Counter1/1, Counter2/1
  Constant6/1 -> Vector FFT1/4
  four_port_gold_code_block1/2(d_out_b) -> Vector Convert5/1
  Constant2/1 -> Relational/1
  Vector Convert2/1 -> Vector Complex Mult2/1(A_re)
  Constant4/1 -> Relational2/2
  Convert1/1 -> Delay5/1, Counter5/1
  Counter4/1 -> Slice2/1
  Vector Convert7/1 -> Vector Complex Mult3/2(A_im)
  Relational4/1 -> Black Box2/2
  Relational/1 -> Subsystem1/2(hold), Subsystem/2(hold)
  Vector Convert6/1 -> Vector Complex Mult2/2(A_im)
  Slice2/1 -> Delay1/1
  four_port_gold_code_block/2(d_out_b) -> Vector Convert1/1
  Vector Convert10/1 -> Subsystem5/5(d1)
  Constant5/1 -> Relational3/2
  Vector Convert3/1 -> Vector Complex Mult3/1(A_re)
  four_port_gold_code_block1/3(d_out_c) -> Vector Convert6/1
  Slice1/1 -> Subsystem2/4(addr_r), Delay/1, Subsystem4/4(addr_r)
  Counter/1 -> Relational1/1, Relational/2
  Subsystem3/1(out) -> Vector FFT1/1
  I.RE/1 -> Vector FFT/1
  Constant1/1 -> Vector FFT/4
  Subsystem1/1(out) -> Subsystem2/2(d)
  four_port_gold_code_block/4(d_out_d) -> Vector Convert3/1
  Vector Convert4/1 -> Vector Complex Mult/2(A_im)
  Counter2/1 -> Relational2/1
  Subsystem4/1(out_A) -> Vector Delay/1

== system full_correlator/Subsystem6 ==
  IN : Inport
  Scalar to Vector2 : hdlSSR/Scalar2Vector  Width=18  sg_ssr=8  block_type=scalar2vector_ssr  XmcBlockStatus=1  sg_ssr_prev=8  maskContainerNames=group1
  Up Sample2 : hdlBasic/Up Sample  sample_ratio=8  copy_samples=on  en=off  latency=1  XmcBlockStatus=1  maskContainerNames=group1  block_type=usamp  block_config=sysgen:Upsample_config
  Vector Reinterpret2 : hdlSSR/Vector Reinterpret  force_arith_type=on  arith_type=Unsigned  force_bin_pt=on  bin_pt=0  sg_ssr=8  block_type=reinterpret_ssr  XmcBlockStatus=1  sg_ssr_prev=8  maskContainerNames=group1
  Vector Reinterpret3 : hdlSSR/Vector Reinterpret  force_arith_type=on  arith_type="Signed  (2's comp)"  force_bin_pt=on  bin_pt=17  sg_ssr=8  block_type=reinterpret_ssr  XmcBlockStatus=1  sg_ssr_prev=8  maskContainerNames=group1
  Vector to Scalar1 : hdlSSR/Vector2Scalar  sg_ssr=8  block_type=vector2scalar_ssr  XmcBlockStatus=1  sg_ssr_prev=8  maskContainerNames=group1
  OUT : Outport
  wires:
  Scalar to Vector2/1 -> Vector Reinterpret3/1
  Vector Reinterpret3/1 -> OUT/1
  Vector Reinterpret2/1 -> Vector to Scalar1/1
  Vector to Scalar1/1 -> Up Sample2/1
  Up Sample2/1 -> Scalar to Vector2/1
  IN/1 -> Vector Reinterpret2/1

== system full_correlator/adc_real_stream ==
  out_reg : Inport
  assert_reg : hdlBasic/Assert  assert_type=on  type_source=Explicitly  gui_display_data_type=Fixed-point  arith_type=Unsigned  n_bits=16  bin_pt=0  preci_type=Single  exp_width=8  frac_width=24  assert_rate=off  rate_source=Explicitly  period=1  output_port=on  XmcBlockStatus=0  maskContainerNames=group1  block_type=assert  block_config=sysgen:assert_config  block_width=609  block_height=900
  cast_gw : hdlBasic/Convert  gui_display_data_type=Fixed-point  arith_type=Unsigned  n_bits=32  bin_pt=0  float_type=Single  exp_bits=8  fraction_bits=24  quantization=Truncate  overflow=Wrap  en=off  latency=1  pipeline=off  XmcBlockStatus=0  maskContainerNames=group2  block_type=convert  block_config=sysgen:Convert_config  block_width=595  block_height=885
  full_correlator_adc_real_stream_user_data_in : hdlBasic/Gateway Out  inherit_from_input=off  hdl_port=on  rows=1  columns=1  UseAsDAC=off  DACChannel='1'  interface=None  automatic_assignment=on  address_offset=hex2dec('00')  intf_name=''  intf_description=''  timing_constraint=None  locs_specified=off  LOCs={}  io_standard={}  XmcBlockStatus=0  maskContainerNames=group4  block_type=gatewayout  block_config=sysgen:gateway_out_config  block_width_w=590  block_height_w=620  block_width=620  block_height=750
  io_delay : hdlBasic/Delay  rst=off  en=off  latency=0  reg_retiming=on  XmcBlockStatus=0  maskContainerNames=group1  block_type=delay  block_config=sysgen:Delay_config
  reint1 : hdlBasic/Reinterpret  force_arith_type=on  arith_type=Unsigned  force_bin_pt=on  bin_pt=0  XmcBlockStatus=0  maskContainerNames=group1  block_type=reinterpret  block_config=sysgen:Reinterpret_config
  sim_out : Terminator
  sim_out_reg_gw : hdlBasic/Gateway Out  inherit_from_input=off  hdl_port=off  rows=1  columns=1  UseAsDAC=off  DACChannel='1'  interface=None  automatic_assignment=on  address_offset=hex2dec('00')  intf_name=''  intf_description=''  timing_constraint=None  locs_specified=off  LOCs={}  io_standard={}  XmcBlockStatus=0  maskContainerNames=group4  block_type=gatewayout  block_config=sysgen:gateway_out_config  block_width_w=590  block_height_w=620  block_width=620  block_height=750
  sim_out_reg_sim_delay : hdlBasic/Delay  rst=off  en=off  latency=1  reg_retiming=on  XmcBlockStatus=0  maskContainerNames=group1  block_type=delay  block_config=sysgen:Delay_config
  sim_out_reg : Outport  VectorParamsAs1DForOutWhenUnconnected=off
  wires:
  sim_out_reg_sim_delay/1 -> sim_out_reg_gw/1
  sim_out_reg_gw/1 -> sim_out_reg/1
  io_delay/1 -> cast_gw/1
  cast_gw/1 -> full_correlator_adc_real_stream_user_data_in/1
  full_correlator_adc_real_stream_user_data_in/1 -> sim_out/1
  out_reg/1 -> sim_out_reg_sim_delay/1, assert_reg/1
  assert_reg/1 -> reint1/1
  reint1/1 -> io_delay/1

== system full_correlator/adc_real_stream1 ==
  out_reg : Inport
  assert_reg : hdlBasic/Assert  assert_type=on  type_source=Explicitly  gui_display_data_type=Fixed-point  arith_type=Unsigned  n_bits=16  bin_pt=0  preci_type=Single  exp_width=8  frac_width=24  assert_rate=off  rate_source=Explicitly  period=1  output_port=on  XmcBlockStatus=0  maskContainerNames=group1  block_type=assert  block_config=sysgen:assert_config  block_width=609  block_height=900
  cast_gw : hdlBasic/Convert  gui_display_data_type=Fixed-point  arith_type=Unsigned  n_bits=32  bin_pt=0  float_type=Single  exp_bits=8  fraction_bits=24  quantization=Truncate  overflow=Wrap  en=off  latency=1  pipeline=off  XmcBlockStatus=0  maskContainerNames=group2  block_type=convert  block_config=sysgen:Convert_config  block_width=595  block_height=885
  full_correlator_adc_real_stream1_user_data_in : hdlBasic/Gateway Out  inherit_from_input=off  hdl_port=on  rows=1  columns=1  UseAsDAC=off  DACChannel='1'  interface=None  automatic_assignment=on  address_offset=hex2dec('00')  intf_name=''  intf_description=''  timing_constraint=None  locs_specified=off  LOCs={}  io_standard={}  XmcBlockStatus=0  maskContainerNames=group4  block_type=gatewayout  block_config=sysgen:gateway_out_config  block_width_w=590  block_height_w=620  block_width=620  block_height=750
  io_delay : hdlBasic/Delay  rst=off  en=off  latency=0  reg_retiming=on  XmcBlockStatus=0  maskContainerNames=group1  block_type=delay  block_config=sysgen:Delay_config
  reint1 : hdlBasic/Reinterpret  force_arith_type=on  arith_type=Unsigned  force_bin_pt=on  bin_pt=0  XmcBlockStatus=0  maskContainerNames=group1  block_type=reinterpret  block_config=sysgen:Reinterpret_config
  sim_out : Terminator
  sim_out_reg_gw : hdlBasic/Gateway Out  inherit_from_input=off  hdl_port=off  rows=1  columns=1  UseAsDAC=off  DACChannel='1'  interface=None  automatic_assignment=on  address_offset=hex2dec('00')  intf_name=''  intf_description=''  timing_constraint=None  locs_specified=off  LOCs={}  io_standard={}  XmcBlockStatus=0  maskContainerNames=group4  block_type=gatewayout  block_config=sysgen:gateway_out_config  block_width_w=590  block_height_w=620  block_width=620  block_height=750
  sim_out_reg_sim_delay : hdlBasic/Delay  rst=off  en=off  latency=1  reg_retiming=on  XmcBlockStatus=0  maskContainerNames=group1  block_type=delay  block_config=sysgen:Delay_config
  sim_out_reg : Outport  VectorParamsAs1DForOutWhenUnconnected=off
  wires:
  sim_out_reg_sim_delay/1 -> sim_out_reg_gw/1
  sim_out_reg_gw/1 -> sim_out_reg/1
  io_delay/1 -> cast_gw/1
  cast_gw/1 -> full_correlator_adc_real_stream1_user_data_in/1
  full_correlator_adc_real_stream1_user_data_in/1 -> sim_out/1
  out_reg/1 -> sim_out_reg_sim_delay/1, assert_reg/1
  assert_reg/1 -> reint1/1
  reint1/1 -> io_delay/1
